simulink model "BLDC_FOC_2"  (R2020a)
settings: Solver=VariableStepAuto  StartTime=0.0  StopTime=10.0  RelTol=1e-3
InitFcn:
  | BLDC_FOC_Params
values from neighbouring files (symbols this model uses):
  J = RotorInertia_KgM2    (= 1.1e-07)    [BLDC_FOC_Params.m]    (also in systemDynamicsFunction.m = evalin('base','J'))
  Ls = PhaseSelfInductance_H    (= 0)    [BLDC_FOC_Params.m]    (also in systemDynamicsFunction.m = evalin('base','Ls'))
  MotorKv = 1890    [BLDC_FOC_Params.m]
  P = MotorPolePairs    (= 4)    [BLDC_FOC_Params.m]    (also in systemDynamicsFunction.m = evalin('base','P'))
undefined symbols (not defined in the file or in its folder): i
libraries: ee_lib x9, nesl_utility x6, eeTransforms x5, simulink x3, fl_lib x2, mcbpositiondecoderlib x1, sharedTrackingLibrary x1
settings Model: Creator=enzoe  LastModifiedBy=enzoe

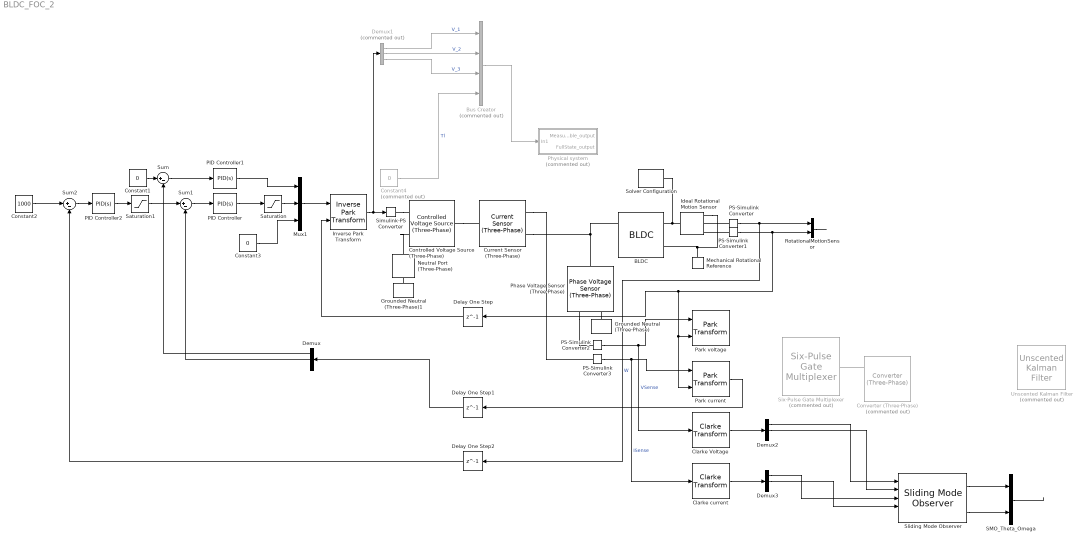
== system BLDC_FOC_2 ==
  BLDC : ee_lib/Electromechanical/Permanent Magnet/BLDC  winding_type=ee.enum.statorconnection.wye  rotor_param=2  pm_flux_linkage=MaximumPermanentMagnetFluxLinkage Wb  theta_constant=(2*pi/3)/P rad  emf_max=MaximumRotorInducedBackEmf_V V  DphiDtheta_tab=[0, -.1528, -.1528, .1528, .1528, 0] Wb/rad  back_emf_tab=[0, -9.6, -9.6, 9.6, 9.6, 0] V  rotor_angle_tab=[0, 7.5, 22.5, 37.5, 52.5, 60] deg  w_meas=RotorSpeedUsedForBackEmfMeasurement_RPM rpm  nPolePairs=P  stator_param=ee.enum.statorparam.LsLmMs  machine_param=ee.enum.dqparameterization.constant  Ld=PhaseInductance H  Lq=PhaseInductance H  idVec=[-200, 0, 200] A  iqVec=[-200, 0, 200] A  LdMatrix=0.00022 * ones(3, 3) H  LqMatrix=0.00022 * ones(3, 3) H  L0=0.00016 H  Ls=Ls H  Lm=0 H  Ms=0 H  Rs=Rs Ohm  zero_sequence=ee.enum.park.zerosequence.include  J=J kg*m^2  lam=B N*m/(rad/s)  axes_param=2  i_d_specify=off  i_d_priority=None  i_d=0 A  i_d_nominal_specify=off  i_d_nominal_unit=A  i_d_nominal_value=1  i_q_specify=off  i_q_priority=None  i_q=0 A  i_q_nominal_specify=off  i_q_nominal_unit=A  i_q_nominal_value=1  torque_specify=off  torque_priority=None  torque=0 N*m  torque_nominal_specify=off  torque_nominal_unit=N*m  torque_nominal_value=1  angular_velocity_specify=off  angular_velocity_priority=High  angular_velocity=0 rpm  angular_velocity_nominal_specify=off  angular_velocity_nominal_unit=rpm  angular_velocity_nominal_value=1  angular_position_specify=off  angular_position_priority=High  angular_position=0 deg  angular_position_nominal_specify=off  angular_position_nominal_unit=deg  angular_position_nominal_value=1  loss_param=ee.enum.ironloss.none  losses_oc=[0, 0, 0] W  losses_sc=[0, 0, 0] W  f_losses=60 Hz  Isc_losses=95 A  Tmeas=298.15 K  alpha=3.93e-3 1/K  alpha_flux=-0.001 1/K  stator_thermal_mass=100 J/K  rotor_thermal_mass=200 J/K  Rm_percent_rotor=90  Rd_percent_rotor=30  temperatureA_specify=off  temperatureA_priority=High  temperatureA=25 degC  temperatureA_nominal_specify=off  temperatureA_nominal_unit=degC  temperatureA_nominal_value=1  temperatureB_specify=off  temperatureB_priority=High  temperatureB=25 degC  temperatureB_nominal_specify=off  temperatureB_nominal_unit=degC  temperatureB_nominal_value=1  temperatureC_specify=off  temperatureC_priority=High  temperatureC=25 degC  temperatureC_nominal_specify=off  temperatureC_nominal_unit=degC  temperatureC_nominal_value=1  temperatureR_specify=off  temperatureR_priority=High  temperatureR=25 degC  temperatureR_nominal_specify=off  temperatureR_nominal_unit=degC  temperatureR_nominal_value=1
      settings: SourceProductBaseCode=PS  InternalSimscapePortConfiguration="{\"Bottom\":[],\"Left\":[{\"id\":\"N\",\"label\":\"~\",\"type\":\"foundation.electrical.three_phase\"},{\"id\":\"n\",\"label\":\"n\",\"type\":\"foundation.electrical.electrical\"}],\"Right\":[{\"id\":\"R\",\"label\":\"R\",\"type\":\"foundation.mechanical.rotational.rotational\"},{\"id\":\"C\",\"label\":\"C\",\"type\":\"foundation.mechanical.rotational.rotational\"}],\"Top\":[]}"
  Bus Creator : BusCreator  Commented=on  Inputs=4
  Clarke Voltage : eeTransforms/Clarke Transform  PowerInvariant=off
      settings: SourceProductBaseCode=PS
  Clarke current : eeTransforms/Clarke Transform  PowerInvariant=off
      settings: SourceProductBaseCode=PS
  Constant1 : Constant  Value=0
  Constant2 : Constant  Value=1000
  Constant3 : Constant  Value=0
  Constant4 : Constant  Commented=on  Value=0
  Controlled Voltage Source (Three-Phase) : ee_lib/Sources/Controlled Voltage Source (Three-Phase)
      settings: SourceProductBaseCode=PS  InternalSimscapePortConfiguration="{\"Bottom\":[],\"Left\":[{\"id\":\"S\",\"label\":\"S\",\"type\":\"input\"},{\"id\":\"n\",\"label\":\"n\",\"type\":\"foundation.electrical.electrical\"}],\"Right\":[{\"id\":\"N\",\"label\":\"~\",\"type\":\"foundation.electrical.three_phase\"}],\"Top\":[]}"
  Converter (Three-Phase) : ee_lib/Semiconductors & Converters/Converters/Converter (Three-Phase)  Commented=on  device_type=ee.enum.converters.switchingdevice.ideal  Vf=0.8 V  Ron=0.001 Ohm  Rds=0.001 Ohm  Goff=1e-6 1/Ohm  Vth=6 V  Vgt=1 V  Vgt_off=-1 V  Ih=1 A  diode_param=ee.enum.converters.protectiondiode.none  diode_Vf=0.8 V  diode_Ron=0.001 Ohm  diode_Goff=1e-5 1/Ohm  diode_C=50 nF  diode_iRM=-235 A  diode_iF=300 A  diode_idot=-50 A/us  diode_trr_param=ee.enum.converters.diodetrr.trr_factor  diode_trr_factor=3  diode_trr=15 us  diode_Qrr=1500 s*uA  snubber_type=ee.enum.converters.snubber.exclude  Rs=0.1 Ohm  Cs=1e-7 F
      settings: SourceProductBaseCode=PS
  Current Sensor (Three-Phase) : ee_lib/Sensors & Transducers/Current Sensor (Three-Phase)
  Delay One Step : Delay  DelayLength=1
  Delay One Step1 : Delay  DelayLength=1
  Delay One Step2 : Delay  DelayLength=1
  Demux : Demux  Outputs=3
  Demux1 : Demux  Commented=on  Outputs=3
  Demux2 : Demux  Outputs=3
  Demux3 : Demux  Outputs=3
  Grounded Neutral (Three-Phase) : ee_lib/Connectors & References/Grounded Neutral (Three-Phase)
      settings: SourceProductBaseCode=PS
  Grounded Neutral (Three-Phase)1 : ee_lib/Connectors & References/Grounded Neutral (Three-Phase)
      settings: SourceProductBaseCode=PS
  Ideal Rotational Motion Sensor : fl_lib/Mechanical/Mechanical Sensors/Ideal Rotational Motion Sensor  wrap_angle=simscape.enum.onoff.on  offset=0 rev
  Inverse Park Transform : eeTransforms/Inverse Park Transform  AxisAlignment=D-axis  PowerInvariant=off
  Mechanical Rotational Reference : fl_lib/Mechanical/Rotational Elements/Mechanical Rotational Reference
  Mux1 : Mux  Inputs=3
  Neutral Port (Three-Phase) : ee_lib/Connectors & References/Neutral Port (Three-Phase)  G_parasitic=1e-12 1/Ohm
      settings: SourceProductBaseCode=PS  InternalSimscapePortConfiguration="{\"Bottom\":[],\"Left\":[{\"id\":\"N\",\"label\":\"~\",\"type\":\"foundation.electrical.three_phase\"}],\"Right\":[{\"id\":\"n\",\"label\":\"n\",\"type\":\"foundation.electrical.electrical\"}],\"Top\":[]}"
  PID Controller : simulink/Continuous/PID Controller  Controller=PID  Form=Parallel  TimeDomain=Continuous-time  UseExternalTs=off  SampleTime=-1  IntegratorMethod=Forward Euler  FilterMethod=Forward Euler  ControllerParametersSource=internal  P=50  I=40  D=0  UseFilter=on  N=100  TunerSelectOption=Transfer Function Based (PID Tuner App)  InitialConditionSource=internal  InitialConditionForIntegrator=0  InitialConditionForFilter=0  DifferentiatorICPrevScaledInput=0  ExternalReset=none  TrackingMode=off  Kt=1  LimitOutput=off  UpperSaturationLimit=inf  LowerSaturationLimit=-inf  LinearizeAsGain=on  AntiWindupMode=none  Kb=1  POutMin=[]  POutMax=[]  IOutMin=[]  IOutMax=[]  DOutMin=[]  DOutMax=[]  NOutMin=[]  NOutMax=[]  SumOutMin=[]  SumOutMax=[]  SaturationOutMin=[]  SaturationOutMax=[]  PParamMin=[]  PParamMax=[]  IParamMin=[]  IParamMax=[]  DParamMin=[]  DParamMax=[]  NParamMin=[]  NParamMax=[]  KbParamMin=[]  KbParamMax=[]  KtParamMin=[]  KtParamMax=[]  KbOutMin=[]  KbOutMax=[]  KtOutMin=[]  KtOutMax=[]  IntegratorOutMin=[]  IntegratorOutMax=[]  FilterOutMin=[]  FilterOutMax=[]  SumI1OutMin=[]  SumI1OutMax=[]  SumI2OutMin=[]  SumI2OutMax=[]  SumI3OutMin=[]  SumI3OutMax=[]  SumI4OutMin=[]  SumI4OutMax=[]  SumDOutMin=[]  SumDOutMax=[]  DifferentiatorOutMin=[]  DifferentiatorOutMax=[]  FilterDiffOutCoefMin=[]  FilterDiffOutCoefMax=[]  ReciprocalOutMin=[]  ReciprocalOutMax=[]  SumDenOutMin=[]  SumDenOutMax=[]  SumNumOutMin=[]  SumNumOutMax=[]  DivideOutMin=[]  DivideOutMax=[]  UdiffTsProdOutMin=[]  UdiffTsProdOutMax=[]  NTsProdOutMin=[]  NTsProdOutMax=[]  UintegralTsProdOutMin=[]  UintegralTsProdOutMax=[]  UngainTsProdOutMin=[]  UngainTsProdOutMax=[]  IntegratorContinuousStateAttributes=''  IntegratorStateMustResolveToSignalObject=off  IntegratorRTWStateStorageClass=Auto  FilterContinuousStateAttributes=''  FilterStateMustResolveToSignalObject=off  FilterRTWStateStorageClass=Auto  ParallelPVariant=InternalParameters  IdealPVariant=Disabled  IVariant=InternalParameters  DVariant=InternalParameters  IntegratorVariant=Continuous  SatVariant=Disabled  AWVariant=Passthrough  PCopyVariant=Disabled  TRVariant=Disabled  FdbkBlocksVariant=Forward  IdealPFdbkVariant=Disabled  SatFdbkVariant=Disabled  DerivativeFilterVariant=ContFilter  NVariant=InternalParameters  NCopyVariant=Disabled  FilterICVariant=InternalICsFilter  IntegratorICVariant=InternalICs  ExternalResetVariant=Disabled  TRSumVariant=Passthrough  SumFdbkVariant=Disabled  SumVariant=Sum_PID  TsampFilterVariant=InternalTs  TsampNgainVariant=Passthrough  TsampIntegralVariant=Passthrough
  PID Controller1 : simulink/Continuous/PID Controller  Controller=PID  Form=Parallel  TimeDomain=Continuous-time  UseExternalTs=off  SampleTime=-1  IntegratorMethod=Forward Euler  FilterMethod=Forward Euler  ControllerParametersSource=internal  P=50  I=40  D=0  UseFilter=on  N=100  TunerSelectOption=Transfer Function Based (PID Tuner App)  InitialConditionSource=internal  InitialConditionForIntegrator=0  InitialConditionForFilter=0  DifferentiatorICPrevScaledInput=0  ExternalReset=none  TrackingMode=off  Kt=1  LimitOutput=off  UpperSaturationLimit=inf  LowerSaturationLimit=-inf  LinearizeAsGain=on  AntiWindupMode=none  Kb=1  POutMin=[]  POutMax=[]  IOutMin=[]  IOutMax=[]  DOutMin=[]  DOutMax=[]  NOutMin=[]  NOutMax=[]  SumOutMin=[]  SumOutMax=[]  SaturationOutMin=[]  SaturationOutMax=[]  PParamMin=[]  PParamMax=[]  IParamMin=[]  IParamMax=[]  DParamMin=[]  DParamMax=[]  NParamMin=[]  NParamMax=[]  KbParamMin=[]  KbParamMax=[]  KtParamMin=[]  KtParamMax=[]  KbOutMin=[]  KbOutMax=[]  KtOutMin=[]  KtOutMax=[]  IntegratorOutMin=[]  IntegratorOutMax=[]  FilterOutMin=[]  FilterOutMax=[]  SumI1OutMin=[]  SumI1OutMax=[]  SumI2OutMin=[]  SumI2OutMax=[]  SumI3OutMin=[]  SumI3OutMax=[]  SumI4OutMin=[]  SumI4OutMax=[]  SumDOutMin=[]  SumDOutMax=[]  DifferentiatorOutMin=[]  DifferentiatorOutMax=[]  FilterDiffOutCoefMin=[]  FilterDiffOutCoefMax=[]  ReciprocalOutMin=[]  ReciprocalOutMax=[]  SumDenOutMin=[]  SumDenOutMax=[]  SumNumOutMin=[]  SumNumOutMax=[]  DivideOutMin=[]  DivideOutMax=[]  UdiffTsProdOutMin=[]  UdiffTsProdOutMax=[]  NTsProdOutMin=[]  NTsProdOutMax=[]  UintegralTsProdOutMin=[]  UintegralTsProdOutMax=[]  UngainTsProdOutMin=[]  UngainTsProdOutMax=[]  IntegratorContinuousStateAttributes=''  IntegratorStateMustResolveToSignalObject=off  IntegratorRTWStateStorageClass=Auto  FilterContinuousStateAttributes=''  FilterStateMustResolveToSignalObject=off  FilterRTWStateStorageClass=Auto  ParallelPVariant=InternalParameters  IdealPVariant=Disabled  IVariant=InternalParameters  DVariant=InternalParameters  IntegratorVariant=Continuous  SatVariant=Disabled  AWVariant=Passthrough  PCopyVariant=Disabled  TRVariant=Disabled  FdbkBlocksVariant=Forward  IdealPFdbkVariant=Disabled  SatFdbkVariant=Disabled  DerivativeFilterVariant=ContFilter  NVariant=InternalParameters  NCopyVariant=Disabled  FilterICVariant=InternalICsFilter  IntegratorICVariant=InternalICs  ExternalResetVariant=Disabled  TRSumVariant=Passthrough  SumFdbkVariant=Disabled  SumVariant=Sum_PID  TsampFilterVariant=InternalTs  TsampNgainVariant=Passthrough  TsampIntegralVariant=Passthrough
  PID Controller2 : simulink/Continuous/PID Controller  Controller=PID  Form=Parallel  TimeDomain=Continuous-time  UseExternalTs=off  SampleTime=-1  IntegratorMethod=Forward Euler  FilterMethod=Forward Euler  ControllerParametersSource=internal  P=0.0003  I=0.0004  D=0  UseFilter=on  N=100  TunerSelectOption=Transfer Function Based (PID Tuner App)  InitialConditionSource=internal  InitialConditionForIntegrator=0  InitialConditionForFilter=0  DifferentiatorICPrevScaledInput=0  ExternalReset=none  TrackingMode=off  Kt=1  LimitOutput=off  UpperSaturationLimit=inf  LowerSaturationLimit=-inf  LinearizeAsGain=on  AntiWindupMode=none  Kb=1  POutMin=[]  POutMax=[]  IOutMin=[]  IOutMax=[]  DOutMin=[]  DOutMax=[]  NOutMin=[]  NOutMax=[]  SumOutMin=[]  SumOutMax=[]  SaturationOutMin=[]  SaturationOutMax=[]  PParamMin=[]  PParamMax=[]  IParamMin=[]  IParamMax=[]  DParamMin=[]  DParamMax=[]  NParamMin=[]  NParamMax=[]  KbParamMin=[]  KbParamMax=[]  KtParamMin=[]  KtParamMax=[]  KbOutMin=[]  KbOutMax=[]  KtOutMin=[]  KtOutMax=[]  IntegratorOutMin=[]  IntegratorOutMax=[]  FilterOutMin=[]  FilterOutMax=[]  SumI1OutMin=[]  SumI1OutMax=[]  SumI2OutMin=[]  SumI2OutMax=[]  SumI3OutMin=[]  SumI3OutMax=[]  SumI4OutMin=[]  SumI4OutMax=[]  SumDOutMin=[]  SumDOutMax=[]  DifferentiatorOutMin=[]  DifferentiatorOutMax=[]  FilterDiffOutCoefMin=[]  FilterDiffOutCoefMax=[]  ReciprocalOutMin=[]  ReciprocalOutMax=[]  SumDenOutMin=[]  SumDenOutMax=[]  SumNumOutMin=[]  SumNumOutMax=[]  DivideOutMin=[]  DivideOutMax=[]  UdiffTsProdOutMin=[]  UdiffTsProdOutMax=[]  NTsProdOutMin=[]  NTsProdOutMax=[]  UintegralTsProdOutMin=[]  UintegralTsProdOutMax=[]  UngainTsProdOutMin=[]  UngainTsProdOutMax=[]  IntegratorContinuousStateAttributes=''  IntegratorStateMustResolveToSignalObject=off  IntegratorRTWStateStorageClass=Auto  FilterContinuousStateAttributes=''  FilterStateMustResolveToSignalObject=off  FilterRTWStateStorageClass=Auto  ParallelPVariant=InternalParameters  IdealPVariant=Disabled  IVariant=InternalParameters  DVariant=InternalParameters  IntegratorVariant=Continuous  SatVariant=Disabled  AWVariant=Passthrough  PCopyVariant=Disabled  TRVariant=Disabled  FdbkBlocksVariant=Forward  IdealPFdbkVariant=Disabled  SatFdbkVariant=Disabled  DerivativeFilterVariant=ContFilter  NVariant=InternalParameters  NCopyVariant=Disabled  FilterICVariant=InternalICsFilter  IntegratorICVariant=InternalICs  ExternalResetVariant=Disabled  TRSumVariant=Passthrough  SumFdbkVariant=Disabled  SumVariant=Sum_PID  TsampFilterVariant=InternalTs  TsampNgainVariant=Passthrough  TsampIntegralVariant=Passthrough
  PS-Simulink Converter{,1..3} (4 alike) : nesl_utility/PS-Simulink Converter  PhysicalDomain=network_engine_domain  SubClassName=ps_output  LeftPortType=input  RightPortType=output  PseudoPeriodic=off  Frequencies=[]  Unit=inherit  AffineConversion=off
  Park current : eeTransforms/Park Transform  AxisAlignment=D-axis  PowerInvariant=off
  Park voltage : eeTransforms/Park Transform  AxisAlignment=D-axis  PowerInvariant=off
  Phase Voltage Sensor (Three-Phase) : ee_lib/Sensors & Transducers/Phase Voltage Sensor (Three-Phase)
      settings: SourceProductBaseCode=PS
  Physical system : Subsystem  Commented=on
  RotationalMotionSensor : Mux  Inputs=2
  SMO_Theta_Omega : Mux  Inputs=2
  Saturation : Saturate  UpperLimit=12  LowerLimit=-12
  Saturation1 : Saturate  UpperLimit=20  LowerLimit=-20
  Simulink-PS Converter : nesl_utility/Simulink-PS Converter  PhysicalDomain=network_engine_domain  SubClassName=ps_input  LeftPortType=input  RightPortType=output  PseudoPeriodic=off  Frequencies=[]  NoiseDistribution=none  NoiseParameters=[]  Unit=1  AffineConversion=off  FilteringAndDerivatives=provide  SimscapeFilterOrder=1  InputFilterTimeConstant=0.001  UdotUserProvided=0
  Six-Pulse Gate Multiplexer : ee_lib/Semiconductors & Converters/Converters/Six-Pulse Gate Multiplexer  Commented=on  R=0 Ohm
      settings: SourceProductBaseCode=PS  InternalSimscapePortConfiguration="{\"Bottom\":[],\"Left\":[{\"id\":\"GaH\",\"label\":\"Ga(H)\",\"type\":\"input\"},{\"id\":\"GaL\",\"label\":\"Ga(L)\",\"type\":\"input\"},{\"id\":\"GbH\",\"label\":\"Gb(H)\",\"type\":\"input\"},{\"id\":\"GbL\",\"label\":\"Gb(L)\",\"type\":\"input\"},{\"id\":\"GcH\",\"label\":\"Gc(H)\",\"type\":\"input\"},{\"id\":\"GcL\",\"label\":\"Gc(L)\",\"type\":\"input\"}],\"Right\":[{\"id\":\"p\",\"label\":\"G\",\"type\":\"foundation.electrical.twelve_phase\"}],\"Top\":[]}"
  Sliding Mode Observer : mcbpositiondecoderlib/Sliding Mode Observer  CurrentObserverGain=0.005  SlidingLimit=2  PositionUnit=Radians  PositionDataType=single  SpeedUnit=RPM  PerUnitSpeed=6000  SpeedDataType=single  BlkSampleTime=50e-6  StatorResistance=Rs  StatorInductance=Ls  MaxApplicationSpeed=MotorKv*12  PolePairs=P  MaxStatorVoltage=12  MaxStatorCurrent=10
      settings: SourceProductBaseCode=MT
  Solver Configuration : nesl_utility/Solver Configuration  PhysicalDomain=network_engine_domain  SubClassName=solver  LeftPortType=input  RightPortType=generic  Tones=[]  Harmonics=[]  SimulateNoise=off  Profile=off  UseLocalSampling=off  EnableSwitchedLinearOptims=on  FrequencyDomain=off  UseCCode=off  RelTol=0.001  AbsTol=1e-06  MinStep=1e-09  ToWorkspace=off  RevertToSquareIcSolve=off  NumHomotopyIterations=100  PhasorMode=off  PhasorModeNumHarmonics=1  DoDC=off  ResidualTolerance=1e-09  UseLocalSolver=on  LocalSolverChoice=NE_BACKWARD_EULER_ADVANCER  LocalSolverSampleTime=1e-5  DoFixedCost=on  MaxNonlinIter=3  MaxModeIter=2  LinearAlgebra=auto  EquationFormulation=NE_TIME_EF  DelaysMemoryBudget=1024  AutomaticFiltering=on  FilteringTimeConstant=0.001  PartitionStorageMethod=AS_NEEDED  PartitionMemoryBudget=1024  PartitionMethod=ROBUST
  Sum : Sum  Inputs=|+-
  Sum1 : Sum  Inputs=|+-
  Sum2 : Sum  Inputs=|+-
  Unscented Kalman Filter : sharedTrackingLibrary/Unscented Kalman Filter  Commented=on  StateTransitionFcn=myStateTransitionFcn  HasAdditiveProcessNoise=Additive  ProcessNoise=1  HasTimeVaryingProcessNoise=off  HasStateTransitionFcnExtraArgument=0  InitialState=0  InitialStateCovariance=1  Alpha=1e-3  Beta=2  Kappa=0  MeasurementFcn1=myMeasurementFcn  HasMeasurementEnablePort1=off  HasAdditiveMeasurementNoise1=Additive  MeasurementNoise1=1  HasTimeVaryingMeasurementNoise1=off  HasMeasurementFcnExtraArgument1=0  MeasurementFcn2=myMeasurementFcn  HasMeasurementEnablePort2=off  HasAdditiveMeasurementNoise2=Additive  MeasurementNoise2=1  HasTimeVaryingMeasurementNoise2=off  HasMeasurementFcnExtraArgument2=0  MeasurementFcn3=myMeasurementFcn  HasMeasurementEnablePort3=off  HasAdditiveMeasurementNoise3=Additive  MeasurementNoise3=1  HasTimeVaryingMeasurementNoise3=off  HasMeasurementFcnExtraArgument3=0  MeasurementFcn4=myMeasurementFcn  HasMeasurementEnablePort4=off  HasAdditiveMeasurementNoise4=Additive  MeasurementNoise4=1  HasTimeVaryingMeasurementNoise4=off  HasMeasurementFcnExtraArgument4=0  MeasurementFcn5=myMeasurementFcn  HasMeasurementEnablePort5=off  HasAdditiveMeasurementNoise5=Additive  MeasurementNoise5=1  HasTimeVaryingMeasurementNoise5=off  HasMeasurementFcnExtraArgument5=0  EnableMultirate=off  StateTransitionFcnSampleTime=1  MeasurementFcn1SampleTime=1  MeasurementFcn2SampleTime=1  MeasurementFcn3SampleTime=1  MeasurementFcn4SampleTime=1  MeasurementFcn5SampleTime=1  UseCurrentEstimator=on  OutputStateCovariance=off  DataType=double  SampleTime=1  NumberOfMeasurements=1
      settings: SourceProductBaseCode=CT,DR,TF,ID,NV,AR,RO,VE
  wires:
  PS-Simulink Converter/1 -> Delay One Step2/1, RotationalMotionSensor/1  "W"
  RotationalMotionSensor/1 -> ?
  PS-Simulink Converter1/1 -> Delay One Step/1, Park current/2, Park voltage/2, RotationalMotionSensor/2
  PS-Simulink Converter2/1 -> Clarke Voltage/1, Park voltage/1  "VSense"
  PS-Simulink Converter3/1 -> Clarke current/1, Park current/1  "ISense"
  Park current/1 -> Delay One Step1/1
  Mux1/1 -> Inverse Park Transform/1
  Clarke Voltage/1 -> Demux2/1
  Clarke current/1 -> Demux3/1
  Constant3/1 -> Mux1/3
  PID Controller1/1 -> Mux1/1
  Sum/1 -> PID Controller1/1
  Constant1/1 -> Sum/1
  Sum1/1 -> PID Controller/1
  PID Controller2/1 -> Saturation1/1
  Demux/1 -> Sum/2
  Demux/2 -> Sum1/2
  Delay One Step1/1 -> Demux/1
  Sum2/1 -> PID Controller2/1
  Constant2/1 -> Sum2/1
  Delay One Step2/1 -> Sum2/2
  Demux1/1 -> Bus Creator/1  "V_1"
  Demux1/3 -> Bus Creator/3  "V_3"
  Demux1/2 -> Bus Creator/2  "V_2"
  Constant4/1 -> Bus Creator/4  "Tl"
  Bus Creator/1 -> Physical system/1(In1)
  Inverse Park Transform/1 -> Demux1/1, Simulink-PS Converter/1
  Delay One Step/1 -> Inverse Park Transform/2
  Demux3/2 -> Sliding Mode Observer/4
  Demux3/1 -> Sliding Mode Observer/3
  Demux2/2 -> Sliding Mode Observer/2
  Demux2/1 -> Sliding Mode Observer/1
  Sliding Mode Observer/1 -> SMO_Theta_Omega/1
  Sliding Mode Observer/2 -> SMO_Theta_Omega/2
  SMO_Theta_Omega/1 -> ?
  PID Controller/1 -> Saturation/1
  Saturation/1 -> Mux1/2
  Saturation1/1 -> Sum1/1
  connections:
  Converter (Three-Phase)/LConn1 -- Six-Pulse Gate Multiplexer/RConn1
  Mechanical Rotational Reference/LConn1 -- Ideal Rotational Motion Sensor/RConn1 -- BLDC/RConn2
  Ideal Rotational Motion Sensor/LConn1 -- Solver Configuration/RConn1 -- BLDC/RConn1
  PS-Simulink Converter/LConn1 -- Ideal Rotational Motion Sensor/RConn2
  PS-Simulink Converter1/LConn1 -- Ideal Rotational Motion Sensor/RConn3
  Phase Voltage Sensor (Three-Phase)/LConn1 -- Current Sensor (Three-Phase)/RConn2 -- BLDC/LConn1
  Grounded Neutral (Three-Phase)/LConn1 -- Phase Voltage Sensor (Three-Phase)/RConn2
  Phase Voltage Sensor (Three-Phase)/RConn1 -- PS-Simulink Converter2/LConn1
  Controlled Voltage Source (Three-Phase)/RConn1 -- Current Sensor (Three-Phase)/LConn1
  Current Sensor (Three-Phase)/RConn1 -- PS-Simulink Converter3/LConn1
  Simulink-PS Converter/RConn1 -- Controlled Voltage Source (Three-Phase)/LConn1
  Controlled Voltage Source (Three-Phase)/LConn2 -- Neutral Port (Three-Phase)/RConn1
  Neutral Port (Three-Phase)/LConn1 -- Grounded Neutral (Three-Phase)1/LConn1

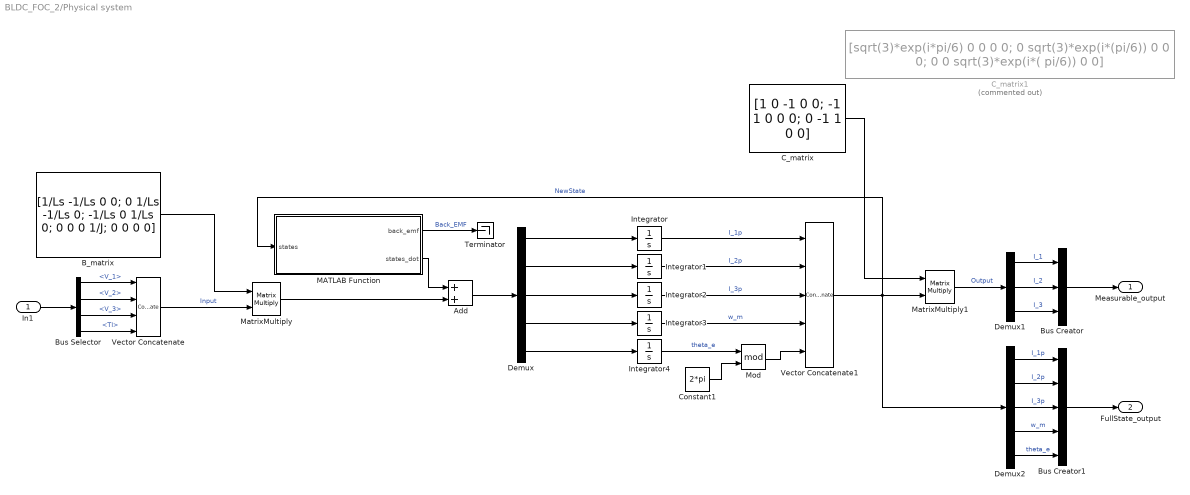
== system BLDC_FOC_2/Physical system ==
  In1 : Inport
  Add : Sum
  B_matrix : Constant  Value=[1/Ls -1/Ls 0 0; 0 1/Ls -1/Ls 0; -1/Ls 0 1/Ls 0; 0 0 0 1/J; 0 0 0 0]
  Bus Creator : BusCreator  Inputs=3
  Bus Creator1 : BusCreator  Inputs=5
  Bus Selector : BusSelector  OutputSignals=V_1,V_2,V_3,Tl
  C_matrix : Constant  Value=[1 0 -1 0 0; -1 1 0 0 0; 0 -1 1 0 0]  VectorParams1D=off
  C_matrix1 : Constant  Commented=on  Value=[sqrt(3)*exp(i*pi/6) 0 0 0 0; 0 sqrt(3)*exp(i*(pi/6)) 0 0 0; 0 0 sqrt(3)*exp(i*( pi/6)) 0 0]  VectorParams1D=off
  Constant1 : Constant  Value=2*pi
  Demux : Demux  Outputs=5
  Demux1 : Demux  Outputs=3
  Demux2 : Demux  Outputs=5
  Integrator{,1..4} (5 alike) : Integrator
  MATLAB Function : MATLAB Function  TreatAsAtomicUnit=on
  MatrixMultiply : Product  Multiplication=Matrix(*)
  MatrixMultiply1 : Product  Multiplication=Matrix(*)
  Mod : Math  Operator=mod  SaturateOnIntegerOverflow=on
  Terminator : Terminator
  Vector Concatenate : Concatenate  NumInputs=4  Mode=Multidimensional array
  Vector Concatenate1 : Concatenate  NumInputs=5  Mode=Multidimensional array
  Measurable_output : Outport
  FullState_output : Outport  Port=2
  wires:
  In1/1 -> Bus Selector/1
  Bus Selector/1 -> Vector Concatenate/1  "<V_1>"
  Bus Selector/2 -> Vector Concatenate/2  "<V_2>"
  Bus Selector/3 -> Vector Concatenate/3  "<V_3>"
  Bus Selector/4 -> Vector Concatenate/4  "<Tl>"
  B_matrix/1 -> MatrixMultiply/1
  Vector Concatenate/1 -> MatrixMultiply/2  "Input"
  Integrator/1 -> Vector Concatenate1/1  "I_1p"
  Integrator1/1 -> Vector Concatenate1/2  "I_2p"
  Integrator2/1 -> Vector Concatenate1/3  "I_3p"
  Integrator3/1 -> Vector Concatenate1/4  "w_m"
  Integrator4/1 -> Mod/1  "theta_e"
  MatrixMultiply/1 -> Add/2
  Add/1 -> Demux/1
  Demux/1 -> Integrator/1
  Demux/2 -> Integrator1/1
  Demux/3 -> Integrator2/1
  Demux/4 -> Integrator3/1
  Demux/5 -> Integrator4/1
  MATLAB Function/2(states_dot) -> Add/1
  Vector Concatenate1/1 -> Demux2/1, MATLAB Function/1(states), MatrixMultiply1/2  "NewState"
  Constant1/1 -> Mod/2
  Mod/1 -> Vector Concatenate1/5
  Bus Creator/1 -> Measurable_output/1
  MatrixMultiply1/1 -> Demux1/1  "Output"
  Demux1/3 -> Bus Creator/3  "I_3"
  Demux1/2 -> Bus Creator/2  "I_2"
  Demux1/1 -> Bus Creator/1  "I_1"
  Bus Creator1/1 -> FullState_output/1
  Demux2/1 -> Bus Creator1/1  "I_1p"
  Demux2/2 -> Bus Creator1/2  "I_2p"
  Demux2/3 -> Bus Creator1/3  "I_3p"
  Demux2/4 -> Bus Creator1/4  "w_m"
  Demux2/5 -> Bus Creator1/5  "theta_e"
  MATLAB Function/1(back_emf) -> Terminator/1  "Back_EMF"
  C_matrix/1 -> MatrixMultiply1/1

== matlab function BLDC_FOC_2/Physical system/MATLAB Function ==
  data: back_emf output; states input; states_dot output size=[5 1]
function [back_emf, states_dot] = SystemDynamics(states)

%#codegen
coder.extrinsic('evalin');
Rs = 0;
Rs = evalin('base','Rs');
Ls = 0;
Ls = evalin('base','Ls');
Ke = 0;
Ke = evalin('base','Ke');
Kt = 0;
Kt = evalin('base','Kt');
J = 0;
J = evalin('base','J');
B = 0;
B = evalin('base','B');
P = 0;
P = evalin('base','P');

%BackEmfGenerator = @BackEmf_sinusoid;
BackEmfGenerator = @BackEmf_Trapezoidal;

A = [-Rs/Ls 0 0 -Ke*BackEmfGenerator(states(5))/Ls 0;
    0 -Rs/Ls 0 -Ke*BackEmfGenerator(states(5) - 2*pi/3)/Ls 0;
    0 0 -Rs/Ls -Ke*BackEmfGenerator(states(5) - 4*pi/3)/Ls 0;
    Kt*BackEmfGenerator(states(5))/J Kt*BackEmfGenerator(states(5) - 2*pi/3)/J Kt*BackEmfGenerator(states(5) - 4*pi/3)/J -B/Ls 0;
    0 0 0 P 0];

back_emf = [Ke*BackEmfGenerator(states(5)) Ke*BackEmfGenerator(states(5) - 2*pi/3) Ke*BackEmfGenerator(states(5) - 4*pi/3)] * states(4);
states_dot = A*states;

end

function BackEmf = BackEmf_Trapezoidal(angle_e_rad)
    if(angle_e_rad < 0)
        angle_e_rad = 2*pi + angle_e_rad;
    end

    % Generate the waveform
    if (0 <= angle_e_rad && angle_e_rad < pi/6)
        BackEmf = angle_e_rad * 6/pi;
    elseif (pi/6 <= angle_e_rad && angle_e_rad < 5*pi/6)
        BackEmf = 1;
    elseif (5*pi/6 <= angle_e_rad && angle_e_rad < 7*pi/6)
        BackEmf = (pi - angle_e_rad) * 6/pi;
    elseif (7*pi/6 <= angle_e_rad && angle_e_rad < 11*pi/6)
        BackEmf = -1;
    elseif (11*pi/6 <= angle_e_rad && angle_e_rad < 2*pi)
        BackEmf = (angle_e_rad - 2*pi) * 6/pi;
    else
        BackEmf = 0;
    end
end

function BackEmf = BackEmf_sinusoid(angle_e_rad)
    BackEmf = sin(angle_e_rad);
end
